simulink model "darko_model"  (R2020b)
settings: Solver=VariableStepAuto  StartTime=0.0  StopTime=1.8  RelTol=1e-3
undefined symbols (not defined in the file or in its folder): x_eq_vol
settings Model: Creator=florian  LastModifiedBy=florian

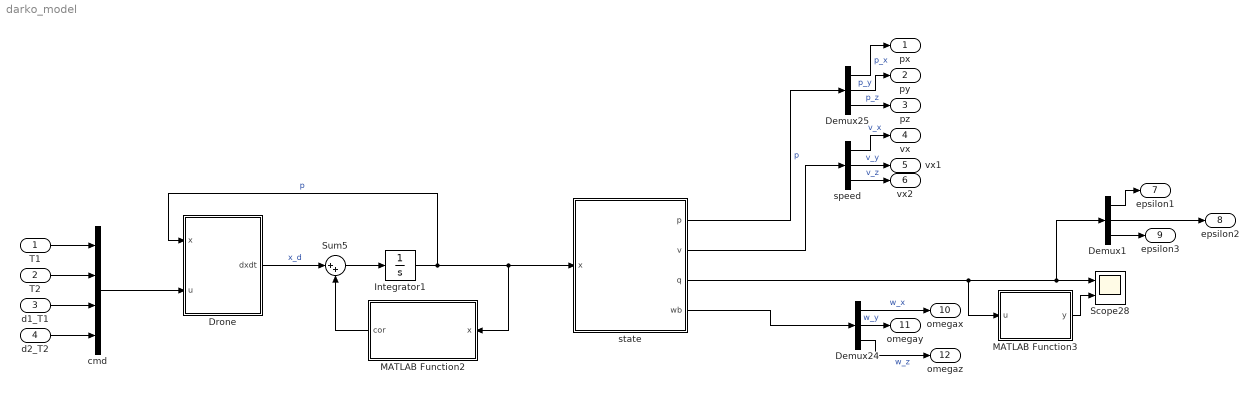
== system darko_model ==
  T1 : Inport
  T2 : Inport  Port=2
  d1_T1 : Inport  Port=3
  d2_T2 : Inport  Port=4
  Demux1 : Demux  Outputs=3
  Demux24 : Demux  Outputs=3
  Demux25 : Demux  Outputs=3
  Drone : MATLAB Function  TreatAsAtomicUnit=on
  Integrator1 : Integrator  InitialCondition=x_eq_vol
  MATLAB Function2 : MATLAB Function  TreatAsAtomicUnit=on
  MATLAB Function3 : MATLAB Function  TreatAsAtomicUnit=on
  Scope28 : Scope  NumInputPorts=2
  Sum5 : Sum  Inputs=|++
  cmd : Mux
  speed : Demux  Outputs=3
  state : MATLAB Function  TreatAsAtomicUnit=on
  px : Outport  VectorParamsAs1DForOutWhenUnconnected=off
  py : Outport  Port=2  VectorParamsAs1DForOutWhenUnconnected=off
  pz : Outport  Port=3  VectorParamsAs1DForOutWhenUnconnected=off
  vx : Outport  Port=4  VectorParamsAs1DForOutWhenUnconnected=off
  vx1 : Outport  Port=5  VectorParamsAs1DForOutWhenUnconnected=off
  vx2 : Outport  Port=6  VectorParamsAs1DForOutWhenUnconnected=off
  epsilon1 : Outport  Port=7  VectorParamsAs1DForOutWhenUnconnected=off
  epsilon2 : Outport  Port=8  VectorParamsAs1DForOutWhenUnconnected=off
  epsilon3 : Outport  Port=9  VectorParamsAs1DForOutWhenUnconnected=off
  omegax : Outport  Port=10  VectorParamsAs1DForOutWhenUnconnected=off
  omegay : Outport  Port=11  VectorParamsAs1DForOutWhenUnconnected=off
  omegaz : Outport  Port=12  VectorParamsAs1DForOutWhenUnconnected=off
  wires:
  Sum5/1 -> Integrator1/1
  MATLAB Function2/1(cor) -> Sum5/2
  Drone/1(dxdt) -> Sum5/1  "x_d"
  Integrator1/1 -> Drone/1(x), state/1(x), MATLAB Function2/1(x)  "p"
  Demux25/3 -> pz/1  "p_z"
  speed/2 -> vx1/1  "v_y"
  Demux24/1 -> omegax/1  "w_x"
  MATLAB Function3/1(y) -> Scope28/2
  state/3(q) -> MATLAB Function3/1(u), Demux1/1, Scope28/1
  Demux25/1 -> px/1  "p_x"
  state/4(wb) -> Demux24/1
  Demux24/2 -> omegay/1  "w_y"
  state/1(p) -> Demux25/1  "p"
  Demux24/3 -> omegaz/1  "w_z"
  state/2(v) -> speed/1
  Demux25/2 -> py/1  "p_y"
  speed/3 -> vx2/1  "v_z"
  speed/1 -> vx/1  "v_x"
  cmd/1 -> Drone/2(u)
  T2/1 -> cmd/2
  T1/1 -> cmd/1
  d1_T1/1 -> cmd/3
  d2_T2/1 -> cmd/4
  Demux1/1 -> epsilon1/1
  Demux1/2 -> epsilon2/1
  Demux1/3 -> epsilon3/1

== matlab function darko_model/Drone ==
  data: x input; u input; dxdt output; drone parameter
function dxdt  = drone(x, u, drone)

%% physical constants
% gravity
g = drone.G;
% vehicle mass
m = drone.MASS;
% vehicle inertia matrix
J = drone.INERTIA; % [3x3 real symmetric] in body axis

%% state demultiplexing
% p = x(1:3);
v = x(4:6);
q  = x(7:10);
wb = x(11:13);

Rq = q2dcm(q);

[Fp, Mp] = external_force_moment(x, u, 0, drone);

% position
dpdt = v;

% kinematics
dvdt =  -[0;0;g] + (1/m)*Rq*drone.Fb*u + (1/m)*Rq*Fp; 

%% quaternion derivative
eta = q(1);
eps = q(2:4);

dqdt = (1/2)*[-eps'; eta*eye(3) + skew_sym(eps)]*wb;

%% angular velocity derivative
% kinematics
dwdt = -J\cross(wb, J*wb) + J\(drone.Mb*u) + J\Mp;


%% derivative multiplexing
dxdt = [dpdt; dvdt; dqdt; dwdt] ;

== matlab function darko_model/MATLAB Function2 ==
  data: x input; cor output
function cor  = fcn(x)
%#codegen
q  = x(7:10);
n = norm(q);
mismatch = 1-n;
cor = [0;0;0; 0;0;0; mismatch*q; 0;0;0];

== matlab function darko_model/MATLAB Function3 ==
  data: u input; y output
function y = fcn(u)
%#codegen

y = norm(u);

== matlab function darko_model/state ==
  data: x input; p output; v output; q output; wb output
function [p, v, q, wb] = demux(x)
%#codegen

p = x(1:3);
v = x(4:6);
q  = x(8:10);
wb = x(11:13);
